simulink model "M2_DAIDALUS"  (R2021a)
settings: Solver=ode4  StartTime=0.0  StopTime=0  RelTol=1e-3
values from neighbouring files (symbols this model uses):
  Intruder = rnfield(Intruder, 'Roll_deg', 'sigma_cross')    [start.m]
undefined symbols (not defined in the file or in its folder): struct2bus
settings Model: Creator=Borshchovi  LastModifiedBy=Borshchovi
settings SolverCC: AlgebraicLoopSolver=TrustRegion
settings DebuggingCC: SFMachineParentedDataDiag=warning
settings SFSimCC: CustomCodeUndefinedFunction=UseInterfaceOnly

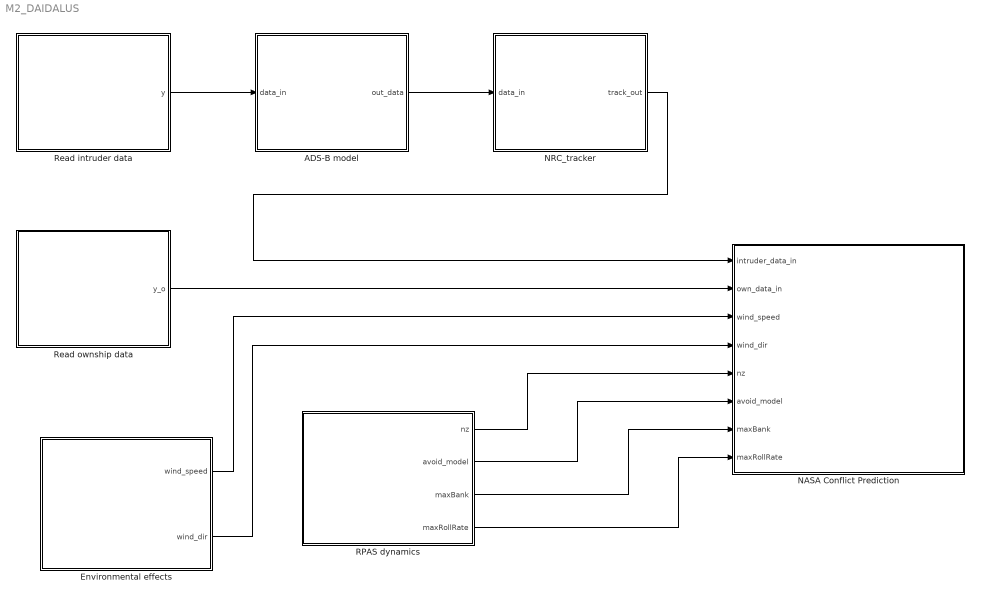
== system M2_DAIDALUS ==
  ADS-B model : MATLAB Function  TreatAsAtomicUnit=on
  Environmental effects : MATLAB Function  TreatAsAtomicUnit=on
  NASA Conflict Prediction : MATLAB Function  TreatAsAtomicUnit=on
  NRC_tracker : MATLAB Function  TreatAsAtomicUnit=on
  RPAS dynamics : MATLAB Function  TreatAsAtomicUnit=on
  Read intruder data : MATLAB Function  InitFcn=struct2bus(Intruder,'mybus')  TreatAsAtomicUnit=on
  Read ownship data : MATLAB Function  InitFcn=struct2bus(Intruder,'mybus')  TreatAsAtomicUnit=on
  wires:
  Read intruder data/1(y) -> ADS-B model/1(data_in)
  ADS-B model/1(out_data) -> NRC_tracker/1(data_in)
  NRC_tracker/1(track_out) -> NASA Conflict Prediction/1(intruder_data_in)
  Read ownship data/1(y_o) -> NASA Conflict Prediction/2(own_data_in)
  Environmental effects/1(wind_speed) -> NASA Conflict Prediction/3(wind_speed)
  Environmental effects/2(wind_dir) -> NASA Conflict Prediction/4(wind_dir)
  RPAS dynamics/1(nz) -> NASA Conflict Prediction/5(nz)
  RPAS dynamics/2(avoid_model) -> NASA Conflict Prediction/6(avoid_model)
  RPAS dynamics/3(maxBank) -> NASA Conflict Prediction/7(maxBank)
  RPAS dynamics/4(maxRollRate) -> NASA Conflict Prediction/8(maxRollRate)

== matlab function M2_DAIDALUS/ADS-B model ==
  data: data_in input; out_data output Bus: mybus
function out_data =ADSB_model(data_in)
% This block supports the Embedded MATLAB subset.
% See the help menu for details. 
% Developed by Iryna B.
   NACp=9;
   count=numel(data_in.GpsTime_s); 
   Time = data_in.GpsTime_s ;
   Lat  =data_in.Lat_deg ;
   Lon  = data_in.Lon_deg ;
   X_cpa=data_in.X_cpa;
   Y_cpa=data_in.Y_cpa;
   Alt  = data_in.Alt_m ; 
   Trk = data_in.Track_deg;
   Spd = data_in.GndSpeed_kts;
   Vz=data_in.Vel_Up_mps;
   Ve = data_in.Vel_E_mps;
   Vn=data_in.Vel_N_mps;
   X=data_in.UTM_E;
   Y=data_in.UTM_N;
   sigma_cross=data_in.sigma_cross;
   sigma_along=data_in.sigma_along;      
  
   timevector=zeros(count,1);
   timevector_late=zeros(count,1);   

   %figure out ADS-B timings
   for i=1:round(count/100)
    timevector(i,1)=data_in.GpsTime_s(1)+i-1;
   end
  
   in_data = struct( 'GpsTime_s', Time,'Lat_deg', Lat, 'Lon_deg', Lon, ...
           'X_cpa',X_cpa,'UTM_E', X, 'UTM_N', Y, 'Alt_m', Alt,'Vel_E_mps', Ve, 'Vel_N_mps', Vn,...
           'Vel_Up_mps', Vz,'GndSpeed_kts', Spd,'Track_deg', Trk, 'Y_cpa',Y_cpa,'sigma_cross', ...
           sigma_cross, 'sigma_along', sigma_along);       

     
   % add noise to position and velocities based on NACp and NACv values
   % DO-282B p.66
   if (NACp==8)
     unc_p = 92.6;
   elseif(NACp==9)
       unc_p = 30;
   elseif(NACp==10)
       unc_p = 10;
   elseif(NACp==11)
       unc_p = 3;
   else
       unc_p = 92.6;
   end
   
  
   % max latency as per DO-282B P.89 Total Latency of Position measurements
   max_latency=0.6;
   laitency = max_latency.*rand(numel(timevector),1)-max_latency; % this ensures the sign being randomly chosen
   timevector_late=timevector+laitency;
   
       
    %Interpolate around those timings 
     
   out_data=Interpolate(in_data, timevector_late); 
  

  
%    shift back the timing 
 
   out_data.GpsTime_s=timevector;

  
   %unc_p is max position uncertainty, which is 4*measurement tolerance
   %(uncertainty), sigma= tolerance/4. use random normally distributed
   %variable to model noise. modeling measurement device systematic error
   %is out of scope  
 
  
   out_data.UTM_E =(normrnd(out_data.UTM_E, sqrt(unc_p)/8,[numel(timevector),1]));
   out_data.UTM_N = (normrnd(out_data.UTM_N, sqrt(unc_p)/8,[numel(timevector),1]));    
   out_data.Alt_m = (normrnd(out_data.Alt_m, unc_p/6,[numel(timevector),1])); %
   
   %First, I thought that estimating velocities from positions was a good
   %idea. apparently I was wrong...Too much noise. Seems like adding noise
   %to truth is a better idea
   out_data.Vel_E_mps= normrnd(out_data.Vel_E_mps, sqrt(unc_p)/64,[numel(timevector),1]);
   out_data.Vel_N_mps= normrnd(out_data.Vel_N_mps, sqrt(unc_p)/64,[numel(timevector),1]);
   out_data.Vel_Up_mps= (normrnd(out_data.Vel_Up_mps, sqrt(unc_p)/64,[numel(timevector),1]));   
    
   out_data.GndSpeed_kts=sqrt(out_data.Vel_E_mps.*out_data.Vel_E_mps+out_data.Vel_N_mps.*out_data.Vel_N_mps);
   out_data.Track_deg=(180/pi*atan2(out_data.Vel_E_mps,out_data.Vel_N_mps));
   
      
   %model resolutions 

   alt_resol=7;  %25 ft  I approximated to 7 m
   out_data.Alt_m=(round(out_data.Alt_m/alt_resol)*alt_resol);
   track_resol=360/256;
   out_data.Track_deg=round(out_data.Track_deg/track_resol)*track_resol;

   speed_resol=1; %1 knot resolution, redundant here
   out_data.GndSpeed_kts=round(out_data.GndSpeed_kts/speed_resol)*speed_resol;
   
   vz_resol=64*0.00508;
   out_data.Vel_Up_mps=(round(out_data.Vel_Up_mps/vz_resol)*vz_resol);
%    
   % Funny is that resolution in horizontal position doesn't affect modeling too much. therefore we roughtly model impact of lat/lon resolution
  
   lat_resol=180/power(2,23)*111000;
   lon_resol=180/power(2,23)*88600;
   out_data.UTM_E=(round(out_data.UTM_E/lon_resol)*lon_resol);
   out_data.UTM_N=(round(out_data.UTM_N/lat_resol)*lat_resol);

== matlab function M2_DAIDALUS/Read intruder data ==
  data: y output Bus: mybus size=1
function y = Read_Intruder_Data
% This block supports the Embedded MATLAB subset.
% See the help menu for details.

% Import MATLAB evalin command
eml.extrinsic('evalin');
% Get contents of the structure a and output it
y = evalin('base', 'Intruder');

== matlab function M2_DAIDALUS/NASA Conflict Prediction ==
  data: intruder_data_in input Bus: mybus; own_data_in input; wind_speed input; wind_dir input; nz input; avoid_model input; maxBank input; maxRollRate input
function DAIDALUS(intruder_data_in,own_data_in, wind_speed, wind_dir, nz, avoid_model, maxBank, maxRollRate)
coder.extrinsic('cd');
coder.extrinsic('DaidalusExample');
coder.extrinsic('disp');

%bring 100 Hz ownship data to 1 Hz
   count=numel(own_data_in.GpsTime_s); 
   Time_o = own_data_in.GpsTime_s ;
   Lat_o  =own_data_in.Lat_deg ;
   Lon_o  = own_data_in.Lon_deg ;
   Alt_o  = own_data_in.Alt_m ; 
   Trk_o = own_data_in.Track_deg;
   Spd_o = own_data_in.GndSpeed_kts;
   Vz_o=own_data_in.Vel_Up_mps;
   Ve_o = own_data_in.Vel_E_mps;
   Vn_o=own_data_in.Vel_N_mps;
   X_o=own_data_in.UTM_E;
   Y_o=own_data_in.UTM_N;
   sigma_cross_o=own_data_in.sigma_cross;
   sigma_along_o=own_data_in.sigma_along;
   X_cpa_o=own_data_in.X_cpa;
   Y_cpa_o=own_data_in.Y_cpa;  
  
   timevector=zeros(count,1);

   %figure out ADS-B timings
   for i=1:round(count/100)
    timevector(i,1)=own_data_in.GpsTime_s(1)+i-1;
   end
  
   own_in_data = struct( 'GpsTime_s', Time_o,'Lat_deg', Lat_o, 'Lon_deg', Lon_o, ...
           'X_cpa', X_cpa_o,'UTM_E', X_o, 'UTM_N', Y_o, 'Alt_m', Alt_o,'Vel_E_mps', Ve_o, 'Vel_N_mps', Vn_o,...
           'Vel_Up_mps', Vz_o,'GndSpeed_kts', Spd_o,'Track_deg', Trk_o, 'Y_cpa',...
           Y_cpa_o, 'sigma_cross', sigma_cross_o, 'sigma_along', sigma_along_o); 
     
   own_out_data=Interpolate(own_in_data, timevector);  

   
   
g=9.80665;
time_resol=1;
override=0; %we override only when needed to manewuver
  
for i=2:round(count/100)
    
     vx_w=wind_speed*sin(wind_dir/180*pi);
     vy_w=wind_speed*cos(wind_dir/180*pi); 
    
     
    
   cd DAIDALUS;


  disp('************************************') ;
   %use DAIDALUS for conflict prediction; This example will not initiate
   %any avoidance maneuver, since DAIDALUS outputs mulptiple maneuvers. The best
   %maneuver to be chosen by the pilot
   %To see the output of DAIDALUS, check Debug->diagnostics window
     DaidalusExample(own_out_data.UTM_E(i), own_out_data.UTM_N(i),own_out_data.Vel_E_mps(i), own_out_data.Vel_N_mps(i),...
             intruder_data_in.UTM_E(i),intruder_data_in.UTM_N(i), intruder_data_in.Vel_E_mps(i),intruder_data_in.Vel_N_mps(i),vx_w, vy_w);  
  cd ..;
  
   
end

== matlab function M2_DAIDALUS/Read ownship data ==
  data: y_o output Bus: mybus size=1
function y_o = Read_Ownship_Data
% This block supports the Embedded MATLAB subset.
% See the help menu for details.

% Import MATLAB evalin command
eml.extrinsic('evalin');
% Get contents of the structure a and output it
y_o = evalin('base', 'Host');

== matlab function M2_DAIDALUS/NRC_tracker ==
  data: data_in input; track_out output Bus: mybus
function track_out=NRC_tracker(data_in)
coder.extrinsic('tracker')
coder.extrinsic('legend')
coder.extrinsic('title')

%because output of the model is samplead for 1 Hz while the actual data before passing
%to model was at 100 Hz
count=round(numel(data_in.UTM_E))/100; 
[X,Y, Vx, Vy, sigma_al, sigma_c]=tracker(data_in.UTM_E, data_in.UTM_N);
% plot(X((1:count),1), Y((1:count),1));
% legend('output');
% hold on

% plot(data_in.UTM_E((1:count),1), data_in.UTM_N((1:count),1));
% legend('detections')
% title('NRC ADS-B tracker');
% grid on;
% hold off

track_out=struct( 'GpsTime_s', data_in.GpsTime_s,'Lat_deg', data_in.Lat_deg, 'Lon_deg', data_in.Lon_deg, ...
            'X_cpa', data_in.X_cpa,'UTM_E', X, 'UTM_N', Y,'Alt_m', data_in.Alt_m,...
            'Vel_E_mps', Vx, 'Vel_N_mps', Vy,'Vel_Up_mps', data_in.Vel_Up_mps,...
            'GndSpeed_kts', data_in.GndSpeed_kts,'Track_deg', data_in.Track_deg, ...
            'Y_cpa', data_in.Y_cpa,'sigma_cross', sigma_c,'sigma_along', sigma_al);

== matlab function M2_DAIDALUS/Environmental effects ==
  data: wind_speed output; wind_dir output
function [wind_speed,wind_dir] =Wind_conditions()
  
wind_speed=10;
wind_dir=-90;

== matlab function M2_DAIDALUS/RPAS dynamics ==
  data: nz output; avoid_model output; maxBank output; maxRollRate output
function [nz,avoid_model, maxBank, maxRollRate] =RPAS_dynamics()
  
nz=1.5; %load factor
avoid_model=1; %use coordinated turn model; 0 if no avoidance  just replay
maxBank = 45;
maxRollRate = 10; % 10 Deg/s roll rate
